simulink subsystem "agent_model_sub"  (R2022b)
settings: Solver=VariableStepAuto  StartTime=0.0  StopTime=10.0  RelTol=1e-3
model mask{InitialCondition=InitialCondition}
  mask prompts: InitialCondition "Simulink:blkprm_prompts:IntegratorInitCond"
values from neighbouring files (symbols this model uses):
  initial_conditions_2 = [6, 3, 2*pi]    [init.m]
settings Model: Creator=gotta  LastModifiedBy=gotta

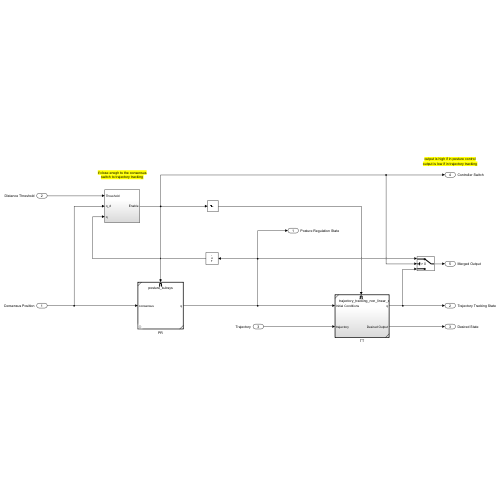
[thumbnail: Simulink's stored preview of the top-level diagram]
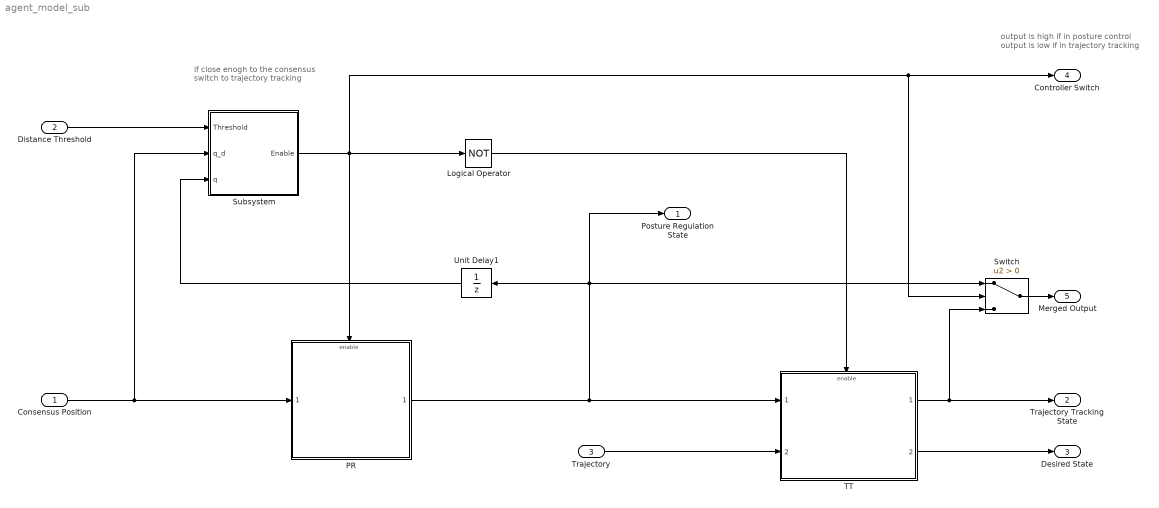
== system agent_model_sub ==
  note: output is high if in posture control
      | output is low if in trajectory tracking
  note: if close enogh to the consensus
      | switch to trajectory tracking
  Consensus Position : Inport
  Distance Threshold : Inport  Port=2
  Trajectory : Inport  Port=3
  Logical Operator : Logic  Operator=NOT  AllPortsSameDT=off  OutDataTypeStr=boolean
  PR : Subsystem  ReferencedSubsystem=posture_subsys  InitialCondition=InitialCondition
  Subsystem : Subsystem
  Switch : Switch  Criteria=u2 > Threshold  SaturateOnIntegerOverflow=off  InputSameDT=off
  TT : Subsystem  ReferencedSubsystem=trajectory_tracking_non_linear_sub
  Unit Delay1 : UnitDelay  InitialCondition=initial_conditions_2  SampleTime=-1  HasFrameUpgradeWarning=on
  Posture Regulation State : Outport
  Trajectory Tracking State : Outport  Port=2
  Desired State : Outport  Port=3
  Controller Switch : Outport  Port=4
  Merged Output : Outport  Port=5
  wires:
  Subsystem/1(Enable) -> Switch/2, Controller Switch/1, Logical Operator/1, PR/Enable
  Switch/1 -> Merged Output/1
  TT/2 -> Desired State/1
  Consensus Position/1 -> PR/1, Subsystem/2(q_d)
  PR/1 -> Switch/1, Posture Regulation State/1, Unit Delay1/1, TT/1
  TT/1 -> Switch/3, Trajectory Tracking State/1
  Unit Delay1/1 -> Subsystem/3(q)
  Logical Operator/1 -> TT/Enable
  Distance Threshold/1 -> Subsystem/1(Threshold)
  Trajectory/1 -> TT/2

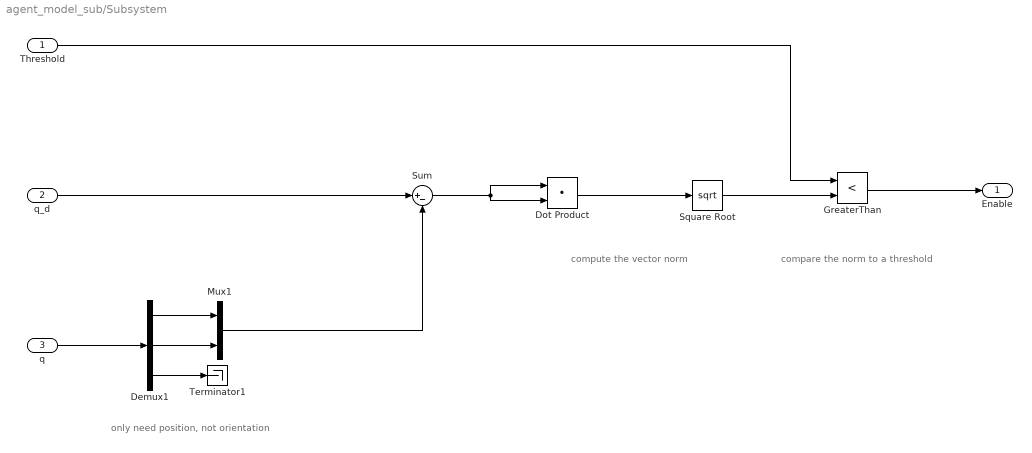
== system agent_model_sub/Subsystem ==
  note: only need position, not orientation
  note: compute the vector norm
  note: compare the norm to a threshold
  Threshold : Inport
  q_d : Inport  Port=2
  q : Inport  Port=3
  Demux1 : Demux  Outputs=3
  Dot Product : DotProduct  OutDataTypeStr=Inherit: Inherit via internal rule
  GreaterThan : RelationalOperator  Operator=<  OutDataTypeStr=boolean  RndMeth=Simplest  InputSameDT=off
  Mux1 : Mux  Inputs=2
  Square Root : Sqrt
  Sum : Sum  Inputs=|+-
  Terminator1 : Terminator
  Enable : Outport
  wires:
  Dot Product/1 -> Square Root/1
  Threshold/1 -> GreaterThan/1
  GreaterThan/1 -> Enable/1
  Sum/1 -> Dot Product/1, Dot Product/2
  Square Root/1 -> GreaterThan/2
  Mux1/1 -> Sum/2
  Demux1/2 -> Mux1/2
  Demux1/3 -> Terminator1/1
  Demux1/1 -> Mux1/1
  q/1 -> Demux1/1
  q_d/1 -> Sum/1
